simulink model "C28069_LLC_ePWM_V8_230307_PhaeShiftWorking"  (R2022b)
settings: Solver=FixedStepAuto  StartTime=0.0  StopTime=10  RelTol=1e-3  EnableMultiTasking=on
model workspace (MAT data in the model file):
  Comp_DAC = 512
undefined symbols (not defined in the file or in its folder): Down, GPTRIP1SEL, GPTRIP2SEL, PWM_Control, PWM_Gen, PWM_Gen1, SCI_A_Transmit, SCI_A_Transmit_Current_Suffix, SCI_A_Transmit_Duty_Suffix, SCI_A_Transmit_Freq_Suffix, SCI_A_Transmit_OVPFlag_Suffix, SCI_A_Transmit_PFC_Suffix, SCI_A_Transmit_SS_Suffix, SCI_A_Transmit_TBPHS_Suffix, SCI_A_Transmit_VADC_Suffix, SCI_A_Transmit_VAvg_Suffix, SCI_A_Transmit_VBAT_Suffix, SCI_A_Transmit_VBATRef_Suffix, SCI_A_Transmit_Vo_Suffix, TZ1, TZ2, u1, Up
libraries: c2802xlib x92, c280xlib x39, simulink x36, c2000lib x1
(part 15 of 18)

== system C28069_LLC_ePWM_V8_230307_PhaeShiftWorking/Softstart @5kHz/GetADC, FaultProtection, SoftStart  @5KHz/UpdatePWM/Frequency Update/Simulink Function1 ==
  note: Original
  note: Frequency Input Selection
  note: Control CMPA/B to Zero
      | When the input is <1KHz
      | (To switch off ePWM)
  note: Fixing deadtime to 250ns
  note: Added Trigger
  PWM_Gen : TriggerPort  TriggerType=function-call  IsSimulinkFunction=on  FunctionName=PWM_Gen  FunctionVisibility=scoped  VariantControl=(inherit)
  CMPA : Display
  CMPA1 : Display
  CMPB : Display
  CMPB1 : Display
  Constant : Constant  Value=100
  Constant1 : Constant
  Constant2 : Constant  Value=0
  Constant3 : Constant  Value=50
  Constant4 : Constant
  Dead time (%) : Display
  Dead time (sec) : Constant  Value=250E-9
  Divide : Product  Inputs=*/
  Gain1 : Gain  Gain=1000
  Gain2 : Gain  Gain=100
  Product{1..4} (4 alike) : Product
  Subsystem1 : Subsystem
  Subtract : Sum  Inputs=+-
  Switch : Switch  Criteria=u2 > Threshold  Threshold=1  SaturateOnIntegerOverflow=off  InputSameDT=off
  Switch1 : Switch  Criteria=u2 > Threshold  OutDataTypeStr=double  SaturateOnIntegerOverflow=off  InputSameDT=off
  TBPRD : Display
  ePWM1 : c2802xlib/ePWM  PwmType=C2000  useModule=ePWM6  ePWMxLINKTBPRD=Not Linked  periodUnits=Clock cycles  timerSource=Input port  timerPeriod_clk=294  timerPeriod_sec=0.0001  tbshadow=Counter equals to zero  countingMode=Up-Down  phaseActiveEnable=Disable  phaseDirection=Count down after sync  phaseActive=0  synchronizationEnable=off  dcaevt1Sync=off  dcbevt1Sync=off  synchronizationOption=Disable  dcbevt1SyncOut=off  dcaevt1SyncOut=off  cmpdSyncOut=off  cmpcSyncOut=off  cmpbSyncOut=off  zeroSyncOut=off  swfSyncOut=off  perSynchronizationOption=Counter equals to period (CTR=PRD)  clockPrescale=1  HSclockPrescale=1  enswap=off  ePWMxAStatus=on  ePWMxAactionLogic1=Do nothing  ePWMxAactionLogic2=Do nothing  ePWMxAactionLogic3=Set  ePWMxAactionLogic4=Do nothing  ePWMxAactionLogic5=Clear  ePWMxAactionLogic6=Do nothing  ePWMxACSFenable=off  ePWMxACSFvalue=Forcing disable  ePWMxASFreload=Zero  ePWMxBStatus=on  ePWMxBactionLogic1=Do nothing  ePWMxBactionLogic2=Do nothing  ePWMxBactionLogic3=Do nothing  ePWMxBactionLogic4=Clear  ePWMxBactionLogic5=Do nothing  ePWMxBactionLogic6=Set  ePWMxBCSFenable=off  ePWMxBCSFvalue=Forcing disable  ePWMxBSFreload=Zero  ePWNxBOutWay=off  ePWMxLINKCMPA=Not Linked  CMPAUnits=Clock cycles  CMPASource=Input port  CMPAValue_per=50  CMPAValue_clk=0  enCMPAshadow=Counter equals to zero (CTR=Zero)  ePWMxLINKCMPB=Not Linked  CMPBUnits=Clock cycles  CMPBSource=Input port  CMPBValue_per=50  CMPBValue_clk=0  enCMPBshadow=Counter equals to zero (CTR=Zero)  ePWMxLINKCMPC=Not Linked  CMPCUnits=Clock cycles  CMPCSource=Specify via dialog  CMPCValue_per=50  CMPCValue_clk=32000  enCMPCshadow=Counter equals to zero (CTR=Zero)  ePWMxLINKCMPD=Not Linked  CMPDUnits=Clock cycles  CMPDSource=Specify via dialog  CMPDValue_per=50  CMPDValue_clk=32000  enCMPDshadow=Counter equals to zero (CTR=Zero)  enableDBePWMxA=off  enableDBePWMxB=off  enhalfcycle=off  DBpolarity=Active high complementary (AHC)  DBedgeDelay=Positive  DBSource_ePWMxA=ePWMxA  DBSource_ePWMxB=ePWMxA  DBPeriodUnits=Clock cycles  DBperiodSource=Input port  REDperiod=10  FEDperiod=10  REDperiod_sec=0  FEDperiod_sec=0  LoadModeDBRED=Immediate without using shadow  LoadModeDBFED=Immediate without using shadow  adcstartModuleA=off  adcrequestEventA=First event  adcstartEventA=Counter equals to zero (CTR=Zero)  adcstartEventA_type2=Digital Compare Module A Event 1 start of conversion (DCAEVT1.soc)  adcstartModuleB=off  adcrequestEventB=First event  adcstartEventB=Counter equals to zero (CTR=Zero)  adcstartEventB_type2=Counter equals to zero (CTR=Zero)  intEn=off  intPrd=First event  intSel=Counter equals to zero (CTR=Zero)  intSel_type2=Counter equals to zero (CTR=Zero)  hrpe=off  enHRPWM=off  HRPWM_LoadMode=Counter equals to period (CTR=PRD)  HRPWM_CTLMode=Duty or Period control mode  HRPWM_EDGMode=Both edge  hrpeb=off  enHRPWMB=off  HRPWM_LoadModeB=Counter equals to zero (CTR=ZERO)  HRPWM_CTLModeB=Duty or Period control mode  HRPWM_EDGModeB=Both edge  enHRDBRED=off  enHRDBFED=off  enSFO=on  enautoconv=on  chopperEnable=off  chopperFrequency=1  chopperFirstwidth=1  chopperDuty=12.5%  tripZonesource=Specify via dialog  tzselOSHT1=off  tzselOSHT2=off  tzselOSHT3=off  tzselOSHDCAEV1=off  tzselOSHDCBEV1=off  tzselCBC1=off  tzselCBC2=off  tzselCBC3=off  tzselCBCDCAEV2=off  tzselCBCDCBEV2=off  tzselOSHT4=off  tzselOSHT5=off  tzselOSHT6=off  tzselCBC4=off  tzselCBC5=off  tzselCBC6=off  enTzOstIntr=off  enTzCbcIntr=off  enTzDCAEVT1Intr=off  enTzDCAEVT2Intr=off  enTzDCBEVT1Intr=off  enTzDCBEVT2Intr=off  ePWMxAforced=No action  ePWMxBforced=No action  DCAEVT1forced=Low  DCBEVT1forced=Low  DCAEVT2forced=No action  DCBEVT2forced=No action  dcah=COMP1OUT input  dcal=Trip Zone 1 input (TZ1)  dcbh=COMP1OUT input  dcbl=Trip Zone 1 input (TZ1)  dcah_type2=GPTRIP1SEL/(TZ1)  dcal_type2=GPTRIP2SEL/(TZ2)  dcbh_type2=GPTRIP1SEL/(TZ1)  dcbl_type2=GPTRIP2SEL/(TZ2)  gendcaevt1=DCAH=high and DCAL=don't care  gendcaevt2=Event disabled  gendcbevt1=DCBH=high and DCBL=don't care  gendcbevt2=Event disabled  dcaevt1src=DCAEVT1 with sync  dcaevt2src=DCAEVT2 with sync  dcbevt1src=DCBEVT1 with sync  dcbevt2src=DCBEVT2 with sync  pulsesel=Counter equals to zero (CTR=Zero)  blankinv=off  blankoffset=0  blankwidth=0  evsrcsel=Filtered version of DCAEVT1 (DCAEVT1FILT)  encape=off
      settings: LibrarySourceBlock=c2806xlib/ePWM
  ePWM4 : c2802xlib/ePWM  PwmType=C2000  useModule=ePWM5  ePWMxLINKTBPRD=Not Linked  periodUnits=Clock cycles  timerSource=Input port  timerPeriod_clk=294  timerPeriod_sec=0.0001  tbshadow=Counter equals to zero  countingMode=Up-Down  phaseActiveEnable=Disable  phaseDirection=Count down after sync  phaseActive=0  synchronizationEnable=off  dcaevt1Sync=off  dcbevt1Sync=off  synchronizationOption=Disable  dcbevt1SyncOut=off  dcaevt1SyncOut=off  cmpdSyncOut=off  cmpcSyncOut=off  cmpbSyncOut=off  zeroSyncOut=off  swfSyncOut=off  perSynchronizationOption=Counter equals to period (CTR=PRD)  clockPrescale=1  HSclockPrescale=1  enswap=off  ePWMxAStatus=on  ePWMxAactionLogic1=Do nothing  ePWMxAactionLogic2=Do nothing  ePWMxAactionLogic3=Set  ePWMxAactionLogic4=Do nothing  ePWMxAactionLogic5=Clear  ePWMxAactionLogic6=Do nothing  ePWMxACSFenable=off  ePWMxACSFvalue=Forcing disable  ePWMxASFreload=Zero  ePWMxBStatus=on  ePWMxBactionLogic1=Do nothing  ePWMxBactionLogic2=Do nothing  ePWMxBactionLogic3=Do nothing  ePWMxBactionLogic4=Clear  ePWMxBactionLogic5=Do nothing  ePWMxBactionLogic6=Set  ePWMxBCSFenable=off  ePWMxBCSFvalue=Forcing disable  ePWMxBSFreload=Zero  ePWNxBOutWay=off  ePWMxLINKCMPA=Not Linked  CMPAUnits=Clock cycles  CMPASource=Input port  CMPAValue_per=50  CMPAValue_clk=0  enCMPAshadow=Counter equals to zero (CTR=Zero)  ePWMxLINKCMPB=Not Linked  CMPBUnits=Clock cycles  CMPBSource=Input port  CMPBValue_per=50  CMPBValue_clk=0  enCMPBshadow=Counter equals to zero (CTR=Zero)  ePWMxLINKCMPC=Not Linked  CMPCUnits=Clock cycles  CMPCSource=Specify via dialog  CMPCValue_per=50  CMPCValue_clk=32000  enCMPCshadow=Counter equals to zero (CTR=Zero)  ePWMxLINKCMPD=Not Linked  CMPDUnits=Clock cycles  CMPDSource=Specify via dialog  CMPDValue_per=50  CMPDValue_clk=32000  enCMPDshadow=Counter equals to zero (CTR=Zero)  enableDBePWMxA=off  enableDBePWMxB=off  enhalfcycle=off  DBpolarity=Active high complementary (AHC)  DBedgeDelay=Positive  DBSource_ePWMxA=ePWMxA  DBSource_ePWMxB=ePWMxA  DBPeriodUnits=Clock cycles  DBperiodSource=Input port  REDperiod=10  FEDperiod=10  REDperiod_sec=0  FEDperiod_sec=0  LoadModeDBRED=Immediate without using shadow  LoadModeDBFED=Immediate without using shadow  adcstartModuleA=on  adcrequestEventA=First event  adcstartEventA=Counter equals to zero (CTR=Zero)  adcstartEventA_type2=Digital Compare Module A Event 1 start of conversion (DCAEVT1.soc)  adcstartModuleB=off  adcrequestEventB=First event  adcstartEventB=Counter equals to zero (CTR=Zero)  adcstartEventB_type2=Counter equals to zero (CTR=Zero)  intEn=on  intPrd=First event  intSel=Counter equals to zero (CTR=Zero)  intSel_type2=Counter equals to zero (CTR=Zero)  hrpe=off  enHRPWM=off  HRPWM_LoadMode=Counter equals to period (CTR=PRD)  HRPWM_CTLMode=Duty or Period control mode  HRPWM_EDGMode=Both edge  hrpeb=off  enHRPWMB=off  HRPWM_LoadModeB=Counter equals to zero (CTR=ZERO)  HRPWM_CTLModeB=Duty or Period control mode  HRPWM_EDGModeB=Both edge  enHRDBRED=off  enHRDBFED=off  enSFO=on  enautoconv=on  chopperEnable=off  chopperFrequency=1  chopperFirstwidth=1  chopperDuty=12.5%  tripZonesource=Specify via dialog  tzselOSHT1=off  tzselOSHT2=off  tzselOSHT3=off  tzselOSHDCAEV1=off  tzselOSHDCBEV1=off  tzselCBC1=off  tzselCBC2=off  tzselCBC3=off  tzselCBCDCAEV2=off  tzselCBCDCBEV2=off  tzselOSHT4=off  tzselOSHT5=off  tzselOSHT6=off  tzselCBC4=off  tzselCBC5=off  tzselCBC6=off  enTzOstIntr=off  enTzCbcIntr=off  enTzDCAEVT1Intr=off  enTzDCAEVT2Intr=off  enTzDCBEVT1Intr=off  enTzDCBEVT2Intr=off  ePWMxAforced=No action  ePWMxBforced=No action  DCAEVT1forced=Low  DCBEVT1forced=Low  DCAEVT2forced=No action  DCBEVT2forced=No action  dcah=COMP1OUT input  dcal=Trip Zone 1 input (TZ1)  dcbh=COMP1OUT input  dcbl=Trip Zone 1 input (TZ1)  dcah_type2=GPTRIP1SEL/(TZ1)  dcal_type2=GPTRIP2SEL/(TZ2)  dcbh_type2=GPTRIP1SEL/(TZ1)  dcbl_type2=GPTRIP2SEL/(TZ2)  gendcaevt1=DCAH=high and DCAL=don't care  gendcaevt2=Event disabled  gendcbevt1=DCBH=high and DCBL=don't care  gendcbevt2=Event disabled  dcaevt1src=DCAEVT1 with sync  dcaevt2src=DCAEVT2 with sync  dcbevt1src=DCBEVT1 with sync  dcbevt2src=DCBEVT2 with sync  pulsesel=Counter equals to zero (CTR=Zero)  blankinv=off  blankoffset=0  blankwidth=0  evsrcsel=Filtered version of DCAEVT1 (DCAEVT1FILT)  encape=off
      settings: LibrarySourceBlock=c2806xlib/ePWM
  original : c2802xlib/ePWM  Commented=on  PwmType=C2000  useModule=ePWM6  ePWMxLINKTBPRD=Not Linked  periodUnits=Clock cycles  timerSource=Input port  timerPeriod_clk=294  timerPeriod_sec=0.0001  tbshadow=Counter equals to zero  countingMode=Up-Down  phaseActiveEnable=Disable  phaseDirection=Count down after sync  phaseActive=0  synchronizationEnable=off  dcaevt1Sync=off  dcbevt1Sync=off  synchronizationOption=Disable  dcbevt1SyncOut=off  dcaevt1SyncOut=off  cmpdSyncOut=off  cmpcSyncOut=off  cmpbSyncOut=off  zeroSyncOut=off  swfSyncOut=off  perSynchronizationOption=Counter equals to period (CTR=PRD)  clockPrescale=1  HSclockPrescale=1  enswap=off  ePWMxAStatus=on  ePWMxAactionLogic1=Do nothing  ePWMxAactionLogic2=Do nothing  ePWMxAactionLogic3=Set  ePWMxAactionLogic4=Do nothing  ePWMxAactionLogic5=Clear  ePWMxAactionLogic6=Do nothing  ePWMxACSFenable=off  ePWMxACSFvalue=Forcing disable  ePWMxASFreload=Zero  ePWMxBStatus=on  ePWMxBactionLogic1=Do nothing  ePWMxBactionLogic2=Do nothing  ePWMxBactionLogic3=Do nothing  ePWMxBactionLogic4=Clear  ePWMxBactionLogic5=Do nothing  ePWMxBactionLogic6=Set  ePWMxBCSFenable=off  ePWMxBCSFvalue=Forcing disable  ePWMxBSFreload=Zero  ePWNxBOutWay=off  ePWMxLINKCMPA=Not Linked  CMPAUnits=Clock cycles  CMPASource=Input port  CMPAValue_per=50  CMPAValue_clk=12  enCMPAshadow=Counter equals to zero (CTR=Zero)  ePWMxLINKCMPB=Not Linked  CMPBUnits=Clock cycles  CMPBSource=Input port  CMPBValue_per=50  CMPBValue_clk=283  enCMPBshadow=Counter equals to zero (CTR=Zero)  ePWMxLINKCMPC=Not Linked  CMPCUnits=Clock cycles  CMPCSource=Specify via dialog  CMPCValue_per=50  CMPCValue_clk=32000  enCMPCshadow=Counter equals to zero (CTR=Zero)  ePWMxLINKCMPD=Not Linked  CMPDUnits=Clock cycles  CMPDSource=Specify via dialog  CMPDValue_per=50  CMPDValue_clk=32000  enCMPDshadow=Counter equals to zero (CTR=Zero)  enableDBePWMxA=off  enableDBePWMxB=off  enhalfcycle=off  DBpolarity=Active high complementary (AHC)  DBedgeDelay=Positive  DBSource_ePWMxA=ePWMxA  DBSource_ePWMxB=ePWMxA  DBPeriodUnits=Clock cycles  DBperiodSource=Input port  REDperiod=10  FEDperiod=10  REDperiod_sec=0  FEDperiod_sec=0  LoadModeDBRED=Immediate without using shadow  LoadModeDBFED=Immediate without using shadow  adcstartModuleA=off  adcrequestEventA=First event  adcstartEventA=Counter equals to zero (CTR=Zero)  adcstartEventA_type2=Digital Compare Module A Event 1 start of conversion (DCAEVT1.soc)  adcstartModuleB=off  adcrequestEventB=First event  adcstartEventB=Counter equals to zero (CTR=Zero)  adcstartEventB_type2=Counter equals to zero (CTR=Zero)  intEn=off  intPrd=First event  intSel=Counter equals to zero (CTR=Zero)  intSel_type2=Counter equals to zero (CTR=Zero)  hrpe=off  enHRPWM=off  HRPWM_LoadMode=Counter equals to period (CTR=PRD)  HRPWM_CTLMode=Duty or Period control mode  HRPWM_EDGMode=Both edge  hrpeb=off  enHRPWMB=off  HRPWM_LoadModeB=Counter equals to zero (CTR=ZERO)  HRPWM_CTLModeB=Duty or Period control mode  HRPWM_EDGModeB=Both edge  enHRDBRED=off  enHRDBFED=off  enSFO=on  enautoconv=on  chopperEnable=off  chopperFrequency=1  chopperFirstwidth=1  chopperDuty=12.5%  tripZonesource=Specify via dialog  tzselOSHT1=off  tzselOSHT2=off  tzselOSHT3=off  tzselOSHDCAEV1=off  tzselOSHDCBEV1=off  tzselCBC1=off  tzselCBC2=off  tzselCBC3=off  tzselCBCDCAEV2=off  tzselCBCDCBEV2=off  tzselOSHT4=off  tzselOSHT5=off  tzselOSHT6=off  tzselCBC4=off  tzselCBC5=off  tzselCBC6=off  enTzOstIntr=off  enTzCbcIntr=off  enTzDCAEVT1Intr=off  enTzDCAEVT2Intr=off  enTzDCBEVT1Intr=off  enTzDCBEVT2Intr=off  ePWMxAforced=No action  ePWMxBforced=No action  DCAEVT1forced=Low  DCBEVT1forced=Low  DCAEVT2forced=No action  DCBEVT2forced=No action  dcah=COMP1OUT input  dcal=Trip Zone 1 input (TZ1)  dcbh=COMP1OUT input  dcbl=Trip Zone 1 input (TZ1)  dcah_type2=GPTRIP1SEL/(TZ1)  dcal_type2=GPTRIP2SEL/(TZ2)  dcbh_type2=GPTRIP1SEL/(TZ1)  dcbl_type2=GPTRIP2SEL/(TZ2)  gendcaevt1=DCAH=high and DCAL=don't care  gendcaevt2=Event disabled  gendcbevt1=DCBH=high and DCBL=don't care  gendcbevt2=Event disabled  dcaevt1src=DCAEVT1 with sync  dcaevt2src=DCAEVT2 with sync  dcbevt1src=DCBEVT1 with sync  dcbevt2src=DCBEVT2 with sync  pulsesel=Counter equals to zero (CTR=Zero)  blankinv=off  blankoffset=0  blankwidth=0  evsrcsel=Filtered version of DCAEVT1 (DCAEVT1FILT)  encape=off
      settings: LibrarySourceBlock=c2806xlib/ePWM
  u : ArgIn  DisableCoverage=on  ArgumentName=u
  wires:
  Constant4/1 -> Switch1/3
  Product4/1 -> ePWM1/3, ePWM4/3, CMPB1/1
  Product3/1 -> CMPA1/1, ePWM4/2, ePWM1/2
  Switch/1 -> Product4/2, Product3/2
  Constant2/1 -> Switch/3
  Constant1/1 -> Switch/1
  Dead time (sec)/1 -> Product1/2
  Gain1/1 -> Product1/1
  Subsystem1/1(Out1) -> TBPRD/1, ePWM1/1, ePWM4/1, Subtract/1, Product2/1
  Product1/1 -> Gain2/1
  Subtract/1 -> CMPB/1, Product4/1
  Constant/1 -> Divide/2
  Product2/1 -> CMPA/1, Product3/1, Subtract/2
  Divide/1 -> Product2/2
  Constant3/1 -> Subsystem1/2(Duty(%))
  u/1 -> Switch1/2, Switch1/1
  Switch1/1 -> Gain1/1, Switch/2, Subsystem1/1(Frequency(kHz))
  Gain2/1 -> Dead time (%)/1, Divide/1

== system C28069_LLC_ePWM_V8_230307_PhaeShiftWorking/Softstart @5kHz/GetADC, FaultProtection, SoftStart  @5KHz/UpdatePWM/Frequency Update/Simulink Function2 ==
  note: Original
  note: Frequency Input Selection
  note: Control CMPA/B to Zero
      | When the input is <1KHz
      | (To switch off ePWM)
  note: Fixing deadtime to 250ns
  note: Added Trigger
  PWM_Gen1 : TriggerPort  TriggerType=function-call  IsSimulinkFunction=on  FunctionName=PWM_Gen1  FunctionVisibility=scoped  VariantControl=(inherit)
  CMPA : Display
  CMPA1 : Display
  CMPB : Display
  CMPB1 : Display
  Constant : Constant  Value=100
  Constant1 : Constant
  Constant2 : Constant  Value=0
  Constant3 : Constant  Value=50
  Constant4 : Constant
  Dead time (%) : Display
  Dead time (sec) : Constant  Value=250E-9
  Divide : Product  Inputs=*/
  Gain1 : Gain  Gain=1000
  Gain2 : Gain  Commented=on  Gain=100
  Product1 : Product  Inputs=3
  Product2 : Product
  Product3 : Product
  Product4 : Product
  Subsystem1 : Subsystem
  Subtract : Sum  Inputs=+-
  Switch : Switch  Criteria=u2 > Threshold  Threshold=1  SaturateOnIntegerOverflow=off  InputSameDT=off
  Switch1 : Switch  Criteria=u2 > Threshold  SaturateOnIntegerOverflow=off  InputSameDT=off
  TBPRD : Display
  ePWM1 : c2802xlib/ePWM  PwmType=C2000  useModule=ePWM6  ePWMxLINKTBPRD=Not Linked  periodUnits=Clock cycles  timerSource=Input port  timerPeriod_clk=294  timerPeriod_sec=0.0001  tbshadow=Counter equals to zero  countingMode=Up-Down  phaseActiveEnable=Disable  phaseDirection=Count down after sync  phaseActive=0  synchronizationEnable=off  dcaevt1Sync=off  dcbevt1Sync=off  synchronizationOption=Disable  dcbevt1SyncOut=off  dcaevt1SyncOut=off  cmpdSyncOut=off  cmpcSyncOut=off  cmpbSyncOut=off  zeroSyncOut=off  swfSyncOut=off  perSynchronizationOption=Counter equals to period (CTR=PRD)  clockPrescale=1  HSclockPrescale=1  enswap=off  ePWMxAStatus=on  ePWMxAactionLogic1=Do nothing  ePWMxAactionLogic2=Do nothing  ePWMxAactionLogic3=Set  ePWMxAactionLogic4=Do nothing  ePWMxAactionLogic5=Clear  ePWMxAactionLogic6=Do nothing  ePWMxACSFenable=off  ePWMxACSFvalue=Forcing disable  ePWMxASFreload=Zero  ePWMxBStatus=on  ePWMxBactionLogic1=Do nothing  ePWMxBactionLogic2=Do nothing  ePWMxBactionLogic3=Do nothing  ePWMxBactionLogic4=Clear  ePWMxBactionLogic5=Do nothing  ePWMxBactionLogic6=Set  ePWMxBCSFenable=off  ePWMxBCSFvalue=Forcing disable  ePWMxBSFreload=Zero  ePWNxBOutWay=off  ePWMxLINKCMPA=Not Linked  CMPAUnits=Clock cycles  CMPASource=Input port  CMPAValue_per=50  CMPAValue_clk=12  enCMPAshadow=Counter equals to zero (CTR=Zero)  ePWMxLINKCMPB=Not Linked  CMPBUnits=Clock cycles  CMPBSource=Input port  CMPBValue_per=50  CMPBValue_clk=283  enCMPBshadow=Counter equals to zero (CTR=Zero)  ePWMxLINKCMPC=Not Linked  CMPCUnits=Clock cycles  CMPCSource=Specify via dialog  CMPCValue_per=50  CMPCValue_clk=32000  enCMPCshadow=Counter equals to zero (CTR=Zero)  ePWMxLINKCMPD=Not Linked  CMPDUnits=Clock cycles  CMPDSource=Specify via dialog  CMPDValue_per=50  CMPDValue_clk=32000  enCMPDshadow=Counter equals to zero (CTR=Zero)  enableDBePWMxA=off  enableDBePWMxB=off  enhalfcycle=off  DBpolarity=Active high complementary (AHC)  DBedgeDelay=Positive  DBSource_ePWMxA=ePWMxA  DBSource_ePWMxB=ePWMxA  DBPeriodUnits=Clock cycles  DBperiodSource=Input port  REDperiod=10  FEDperiod=10  REDperiod_sec=0  FEDperiod_sec=0  LoadModeDBRED=Immediate without using shadow  LoadModeDBFED=Immediate without using shadow  adcstartModuleA=off  adcrequestEventA=First event  adcstartEventA=Counter equals to zero (CTR=Zero)  adcstartEventA_type2=Digital Compare Module A Event 1 start of conversion (DCAEVT1.soc)  adcstartModuleB=off  adcrequestEventB=First event  adcstartEventB=Counter equals to zero (CTR=Zero)  adcstartEventB_type2=Counter equals to zero (CTR=Zero)  intEn=off  intPrd=First event  intSel=Counter equals to zero (CTR=Zero)  intSel_type2=Counter equals to zero (CTR=Zero)  hrpe=off  enHRPWM=off  HRPWM_LoadMode=Counter equals to period (CTR=PRD)  HRPWM_CTLMode=Duty or Period control mode  HRPWM_EDGMode=Both edge  hrpeb=off  enHRPWMB=off  HRPWM_LoadModeB=Counter equals to zero (CTR=ZERO)  HRPWM_CTLModeB=Duty or Period control mode  HRPWM_EDGModeB=Both edge  enHRDBRED=off  enHRDBFED=off  enSFO=on  enautoconv=on  chopperEnable=off  chopperFrequency=1  chopperFirstwidth=1  chopperDuty=12.5%  tripZonesource=Specify via dialog  tzselOSHT1=off  tzselOSHT2=off  tzselOSHT3=off  tzselOSHDCAEV1=off  tzselOSHDCBEV1=off  tzselCBC1=off  tzselCBC2=off  tzselCBC3=off  tzselCBCDCAEV2=off  tzselCBCDCBEV2=off  tzselOSHT4=off  tzselOSHT5=off  tzselOSHT6=off  tzselCBC4=off  tzselCBC5=off  tzselCBC6=off  enTzOstIntr=off  enTzCbcIntr=off  enTzDCAEVT1Intr=off  enTzDCAEVT2Intr=off  enTzDCBEVT1Intr=off  enTzDCBEVT2Intr=off  ePWMxAforced=No action  ePWMxBforced=No action  DCAEVT1forced=Low  DCBEVT1forced=Low  DCAEVT2forced=No action  DCBEVT2forced=No action  dcah=COMP1OUT input  dcal=Trip Zone 1 input (TZ1)  dcbh=COMP1OUT input  dcbl=Trip Zone 1 input (TZ1)  dcah_type2=GPTRIP1SEL/(TZ1)  dcal_type2=GPTRIP2SEL/(TZ2)  dcbh_type2=GPTRIP1SEL/(TZ1)  dcbl_type2=GPTRIP2SEL/(TZ2)  gendcaevt1=DCAH=high and DCAL=don't care  gendcaevt2=Event disabled  gendcbevt1=DCBH=high and DCBL=don't care  gendcbevt2=Event disabled  dcaevt1src=DCAEVT1 with sync  dcaevt2src=DCAEVT2 with sync  dcbevt1src=DCBEVT1 with sync  dcbevt2src=DCBEVT2 with sync  pulsesel=Counter equals to zero (CTR=Zero)  blankinv=off  blankoffset=0  blankwidth=0  evsrcsel=Filtered version of DCAEVT1 (DCAEVT1FILT)  encape=off
      settings: LibrarySourceBlock=c2806xlib/ePWM
  ePWM4 : c2802xlib/ePWM  PwmType=C2000  useModule=ePWM5  ePWMxLINKTBPRD=Not Linked  periodUnits=Clock cycles  timerSource=Input port  timerPeriod_clk=294  timerPeriod_sec=0.0001  tbshadow=Counter equals to zero  countingMode=Up-Down  phaseActiveEnable=Disable  phaseDirection=Count down after sync  phaseActive=0  synchronizationEnable=off  dcaevt1Sync=off  dcbevt1Sync=off  synchronizationOption=Disable  dcbevt1SyncOut=off  dcaevt1SyncOut=off  cmpdSyncOut=off  cmpcSyncOut=off  cmpbSyncOut=off  zeroSyncOut=off  swfSyncOut=off  perSynchronizationOption=Counter equals to period (CTR=PRD)  clockPrescale=1  HSclockPrescale=1  enswap=off  ePWMxAStatus=on  ePWMxAactionLogic1=Do nothing  ePWMxAactionLogic2=Do nothing  ePWMxAactionLogic3=Set  ePWMxAactionLogic4=Do nothing  ePWMxAactionLogic5=Clear  ePWMxAactionLogic6=Do nothing  ePWMxACSFenable=off  ePWMxACSFvalue=Forcing disable  ePWMxASFreload=Zero  ePWMxBStatus=on  ePWMxBactionLogic1=Do nothing  ePWMxBactionLogic2=Do nothing  ePWMxBactionLogic3=Do nothing  ePWMxBactionLogic4=Clear  ePWMxBactionLogic5=Do nothing  ePWMxBactionLogic6=Set  ePWMxBCSFenable=off  ePWMxBCSFvalue=Forcing disable  ePWMxBSFreload=Zero  ePWNxBOutWay=off  ePWMxLINKCMPA=Not Linked  CMPAUnits=Clock cycles  CMPASource=Input port  CMPAValue_per=50  CMPAValue_clk=12  enCMPAshadow=Counter equals to zero (CTR=Zero)  ePWMxLINKCMPB=Not Linked  CMPBUnits=Clock cycles  CMPBSource=Input port  CMPBValue_per=50  CMPBValue_clk=283  enCMPBshadow=Counter equals to zero (CTR=Zero)  ePWMxLINKCMPC=Not Linked  CMPCUnits=Clock cycles  CMPCSource=Specify via dialog  CMPCValue_per=50  CMPCValue_clk=32000  enCMPCshadow=Counter equals to zero (CTR=Zero)  ePWMxLINKCMPD=Not Linked  CMPDUnits=Clock cycles  CMPDSource=Specify via dialog  CMPDValue_per=50  CMPDValue_clk=32000  enCMPDshadow=Counter equals to zero (CTR=Zero)  enableDBePWMxA=off  enableDBePWMxB=off  enhalfcycle=off  DBpolarity=Active high complementary (AHC)  DBedgeDelay=Positive  DBSource_ePWMxA=ePWMxA  DBSource_ePWMxB=ePWMxA  DBPeriodUnits=Clock cycles  DBperiodSource=Input port  REDperiod=10  FEDperiod=10  REDperiod_sec=0  FEDperiod_sec=0  LoadModeDBRED=Immediate without using shadow  LoadModeDBFED=Immediate without using shadow  adcstartModuleA=on  adcrequestEventA=First event  adcstartEventA=Counter equals to zero (CTR=Zero)  adcstartEventA_type2=Digital Compare Module A Event 1 start of conversion (DCAEVT1.soc)  adcstartModuleB=off  adcrequestEventB=First event  adcstartEventB=Counter equals to zero (CTR=Zero)  adcstartEventB_type2=Counter equals to zero (CTR=Zero)  intEn=on  intPrd=First event  intSel=Counter equals to zero (CTR=Zero)  intSel_type2=Counter equals to zero (CTR=Zero)  hrpe=off  enHRPWM=off  HRPWM_LoadMode=Counter equals to period (CTR=PRD)  HRPWM_CTLMode=Duty or Period control mode  HRPWM_EDGMode=Both edge  hrpeb=off  enHRPWMB=off  HRPWM_LoadModeB=Counter equals to zero (CTR=ZERO)  HRPWM_CTLModeB=Duty or Period control mode  HRPWM_EDGModeB=Both edge  enHRDBRED=off  enHRDBFED=off  enSFO=on  enautoconv=on  chopperEnable=off  chopperFrequency=1  chopperFirstwidth=1  chopperDuty=12.5%  tripZonesource=Specify via dialog  tzselOSHT1=off  tzselOSHT2=off  tzselOSHT3=off  tzselOSHDCAEV1=off  tzselOSHDCBEV1=off  tzselCBC1=off  tzselCBC2=off  tzselCBC3=off  tzselCBCDCAEV2=off  tzselCBCDCBEV2=off  tzselOSHT4=off  tzselOSHT5=off  tzselOSHT6=off  tzselCBC4=off  tzselCBC5=off  tzselCBC6=off  enTzOstIntr=off  enTzCbcIntr=off  enTzDCAEVT1Intr=off  enTzDCAEVT2Intr=off  enTzDCBEVT1Intr=off  enTzDCBEVT2Intr=off  ePWMxAforced=No action  ePWMxBforced=No action  DCAEVT1forced=Low  DCBEVT1forced=Low  DCAEVT2forced=No action  DCBEVT2forced=No action  dcah=COMP1OUT input  dcal=Trip Zone 1 input (TZ1)  dcbh=COMP1OUT input  dcbl=Trip Zone 1 input (TZ1)  dcah_type2=GPTRIP1SEL/(TZ1)  dcal_type2=GPTRIP2SEL/(TZ2)  dcbh_type2=GPTRIP1SEL/(TZ1)  dcbl_type2=GPTRIP2SEL/(TZ2)  gendcaevt1=DCAH=high and DCAL=don't care  gendcaevt2=Event disabled  gendcbevt1=DCBH=high and DCBL=don't care  gendcbevt2=Event disabled  dcaevt1src=DCAEVT1 with sync  dcaevt2src=DCAEVT2 with sync  dcbevt1src=DCBEVT1 with sync  dcbevt2src=DCBEVT2 with sync  pulsesel=Counter equals to zero (CTR=Zero)  blankinv=off  blankoffset=0  blankwidth=0  evsrcsel=Filtered version of DCAEVT1 (DCAEVT1FILT)  encape=off
      settings: LibrarySourceBlock=c2806xlib/ePWM
  u : ArgIn  DisableCoverage=on  OutDataTypeStr=uint16  ArgumentName=u
  u1 : ArgIn  DisableCoverage=on  Port=2  OutDataTypeStr=uint16  ArgumentName=u1
  wires:
  Constant4/1 -> Switch1/3
  Product4/1 -> ePWM1/3, ePWM4/3, CMPB1/1
  Product3/1 -> CMPA1/1, ePWM4/2, ePWM1/2
  Switch/1 -> Product4/2, Product3/2
  Constant2/1 -> Switch/3
  Constant1/1 -> Switch/1
  Dead time (sec)/1 -> Product1/2
  Gain1/1 -> Product1/1
  Subsystem1/1(Out1) -> TBPRD/1, ePWM1/1, ePWM4/1, Subtract/1, Product2/1
  Product1/1 -> Dead time (%)/1, Divide/1
  Subtract/1 -> CMPB/1, Product4/1
  Constant/1 -> Divide/2
  Product2/1 -> CMPA/1, Product3/1, Subtract/2
  Divide/1 -> Product2/2
  Constant3/1 -> Subsystem1/2(Duty(%))
  u/1 -> Switch1/2, Switch1/1
  Switch1/1 -> Gain1/1, Switch/2, Subsystem1/1(Frequency(kHz))
  u1/1 -> Product1/3

== system C28069_LLC_ePWM_V8_230307_PhaeShiftWorking/Softstart @5kHz/GetADC, FaultProtection, SoftStart  @5KHz/UpdatePWM/Frequency Update/Simulink Function1/Subsystem1 ==
  Frequency(kHz) : Inport  OutDataTypeStr=double
  Duty(%) : Inport  Port=2
  Constant1 : Constant  Value=90E6
  Divide : Product  Inputs=*/  RndMeth=Zero  SaturateOnIntegerOverflow=on
  Gain : Gain  Gain=1000
  Gain1 : Gain  Gain=1/100
  Gain2 : Gain  Gain=0.5
  Product : Product
  Product1 : Product
  Up-Down Counter : Constant  Value=2
  Out1 : Outport
  Out2 : Outport  Port=2
  Out3 : Outport  Port=3
  wires:
  Gain2/1 -> Out3/1
  Gain1/1 -> Product1/2
  Product1/1 -> Gain2/1, Out2/1
  Duty(%)/1 -> Gain1/1
  Divide/1 -> Out1/1, Product1/1
  Constant1/1 -> Divide/1
  Frequency(kHz)/1 -> Gain/1
  Product/1 -> Divide/2
  Gain/1 -> Product/1
  Up-Down Counter/1 -> Product/2

== system C28069_LLC_ePWM_V8_230307_PhaeShiftWorking/Softstart @5kHz/GetADC, FaultProtection, SoftStart  @5KHz/UpdatePWM/Frequency Update/Simulink Function2/Subsystem1 ==
  Frequency(kHz) : Inport
  Duty(%) : Inport  Port=2
  Constant1 : Constant  Value=90E6
  Divide : Product  Inputs=*/  RndMeth=Zero  SaturateOnIntegerOverflow=on
  Gain : Gain  Gain=1000
  Gain1 : Gain  Gain=1/100
  Gain2 : Gain  Gain=0.5
  Product : Product
  Product1 : Product
  Up-Down Counter : Constant  Value=2
  Out1 : Outport
  Out2 : Outport  Port=2
  Out3 : Outport  Port=3
  wires:
  Gain2/1 -> Out3/1
  Gain1/1 -> Product1/2
  Product1/1 -> Gain2/1, Out2/1
  Duty(%)/1 -> Gain1/1
  Divide/1 -> Out1/1, Product1/1
  Constant1/1 -> Divide/1
  Frequency(kHz)/1 -> Gain/1
  Product/1 -> Divide/2
  Gain/1 -> Product/1
  Up-Down Counter/1 -> Product/2

== stateflow chart C28069_LLC_ePWM_V8_230307_PhaeShiftWorking/GetADC, FaultProtection, SoftStart  @5KHz/UpdatePWM1/SoftStart/If Action Subsystem/ReservseSoftStart1/Chart1 ==
  note: Under 5KHz, 1 = 0.0002s/cycle
      | 1000 = 0.2s per increment/decrement
  note: [Frequency_Adjusted == Resonant_Frequency]
      | will go here
  note: To initialise the frequency
  note: For increment of 110 (+-5% each DC)
      | Duty_Adjusted @ 660 = 15% Duty
      | '' @ 770 = 10% Duty
      | - - - - - - - - - - - - - - - -
      | 715 + 55 = 15% DutyCycle
      | 660 + 55 (+-2.5%DC) = ~18% DutyCycle = 1us (Minimum required)
  (default) -> (junction 47)
  (junction 47) -> (junction 62) [order 2]
  (junction 62) -> (junction 64) : {
      | First_Pass = 1;
      | Soft_Start = 1;
      | Local_counter = 1;
      | SoftStart_OK = 0;
      | Duty_Adjusted = 100;
      | }
  (junction 47) -> (junction 48) [order 1] : [PFC_OK]
  (junction 48) -> (junction 49) [order 1] : [First_Pass]
  (junction 48) -> (junction 56) [order 2] : [Soft_Start]
  (junction 56) -> (junction 58) [order 1] : [Local_counter > 600]
      | {
      | Local_counter = 0;
      | }
  (junction 58) -> (junction 74) [order 2]
  (junction 74) -> (junction 81) [order 1] : [abs(Frequency_Adjusted - Resonant_Frequency)<1]
  (junction 48) -> (junction 105) [order 4]
  (junction 49) -> (junction 60) : {
      | Frequency_Adjusted = Initial_Frequency;
      | First_Pass = 0;
      | }
  (junction 48) -> (junction 102) [order 3] : [Duty_Adjusted <= 550]
  (junction 56) -> (junction 70) [order 2] : {
      | Local_counter = Local_counter +1;
      | }
  (junction 58) -> (junction 68) [order 1] : [Frequency_Adjusted > Resonant_Frequency]
      | {
      | Frequency_Adjusted = Frequency_Adjusted - 0.1;
      | }
  (junction 74) -> (junction 76) [order 2] : [Frequency_Adjusted < Resonant_Frequency]
      |
      | {
      | Frequency_Adjusted = Frequency_Adjusted + 0.1;
      | }
  (junction 81) -> (junction 84) : {
      | SoftStart_OK = 1;
      | Soft_Start = 0;
      | %%Frequency_Adjusted = Initial_Frequency;
      | }
  (junction 102) -> (junction 105) [order 2] : {
      | Local_counter = Local_counter +1;
      | }
  (junction 105) -> (junction 51)
  (junction 102) -> (junction 108) [order 1] : [Local_counter >600]
      | {
      | Local_counter = 0;
      | }
  (junction 108) -> (junction 51) : {
      | Duty_Adjusted = Duty_Adjusted + 55;
      | }
  (junction 64) -> (junction 60)
  (junction 60) -> (junction 51)
  (junction 51) -> (junction 70)
  (junction 70) -> (junction 68)
  (junction 68) -> (junction 76)
  (junction 84) -> (junction 76)
  data: SoftStart_OK output; Duty_Adjusted output =100; PFC_OK input; Initial_Frequency input; Resonant_Frequency input; Local_counter local =1; Frequency_Adjusted output double; First_Pass local =1; Soft_Start local =1

== stateflow chart C28069_LLC_ePWM_V8_230307_PhaeShiftWorking/GetADC, FaultProtection, SoftStart  @5KHz/UpdatePWM1/SoftStart/If Action Subsystem/SoftStart1/Chart ==
  note: Verror = Vbulk_Ref_ADC_adjusted - Vbulk_ADC;
  note: Local variables
      | VbusRefTemp
      | SoftStartCnt
  (default) -> (junction 47)
  (junction 47) -> (junction 50) [order 2]
  (junction 50) -> (junction 52) : {
      | First_Pass=1;
      | Soft_Start=1;
      | SoftStartCnt=1;
      | %Debug=1;
      | }
  (junction 47) -> (junction 5) [order 1] : [PFC_OK]
  (junction 5) -> (junction 7) [order 1] : [First_Pass]
  (junction 5) -> (junction 15) [order 2] : [Soft_Start]
  (junction 15) -> (junction 18) [order 1] : [SoftStartCnt>100]
      | %% At every 5 cycles (total 1ms),
  (junction 18) -> (junction 23) [order 2] : %{Debug=Vbulk_Ref_ADC_adjusted;}
  (junction 23) -> (junction 31) : %{Debug=6;}
  (junction 31) -> (junction 55) [commented out] : [abs(VBAT_Ref_adjusted - VBAT_Ref)<1]
  (junction 7) -> (junction 10) : {
      | VBAT_Ref_adjusted = VBAT_Value;
      | %Vbulk_Ref_ADC_adjusted = Vbulk_Ref_ADC;
      | First_Pass = 0;
      | %Debug=2;
      |
      | }
  (junction 5) -> (junction 38) [order 3] : {
      | SoftStart_OK = 1;
      | %Debug=3;
      | %Vbulk_Ref_ADC_adjusted=Vbulk_Ref_ADC;
      | }
  (junction 15) -> (junction 20) [order 2] : {
      | SoftStartCnt = SoftStartCnt + 1;
      | %Debug=4;
      | }
      | %% incerase the counter first.
  (junction 18) -> (junction 64) [order 1] : [VBAT_Ref_adjusted < VBAT_Ref]
      | {VBAT_Ref_adjusted = VBAT_Ref_adjusted + 0.1;}
      | %% Increase the reference voltage
  (junction 23) -> (junction 26) [commented out] : [VBAT_Ref_adjusted > VBAT_Ref]
      | {VBAT_Ref_adjusted = VBAT_Ref_adjusted - 0.1;
      | }
      | %% Reduce the reference voltage
  (junction 31) -> (junction 33) : {
      | Soft_Start=0;
      | SoftStartCnt=0;
      | %Debug=7;
      | VBAT_Ref_adjusted=VBAT_Ref;
      | }
      | %% End soft start
  (junction 55) -> (junction 57) [commented out] : {
      | Soft_Start=0;
      | SoftStartCnt=0;
      | VBAT_Ref_adjusted=VBAT_Ref;
      | %Debug=8;
      | }
  (junction 64) -> (junction 28) [order 2]
  (junction 64) -> (junction 28) [order 1] : [VBAT_Ref_adjusted < VBAT_Value]
      | {VBAT_Ref_adjusted = VBAT_Value ;}
      | %% Increase the reference voltage
  (junction 52) -> (junction 10)
  (junction 10) -> (junction 38)
  (junction 26) -> (junction 28)
  (junction 33) -> (junction 26)
  (junction 57) -> (junction 33) [commented out]
  (junction 20) -> (junction 38)
  (junction 28) -> (junction 20)
  data: PFC_OK input; VBAT_Value input; VbusRefTemp local =0; SoftStartCnt local =0; VBAT_Ref input double; VBAT_Ref_adjusted output double =0; Vbulk_Ref_ADC_Hard_Value local =0; First_Pass1 local; First_Pass local =1; Soft_Start local =1; SoftStart_OK output

== stateflow chart C28069_LLC_ePWM_V8_230307_PhaeShiftWorking/GetADC, FaultProtection, SoftStart  @5KHz/UpdatePWM1/SoftStart/If Action Subsystem/SoftStart1/Chart1 ==
  note: Under 5KHz, 1 = 0.0002s/cycle
      | 1000 = 0.2s per increment/decrement
  note: [Frequency_Adjusted == Resonant_Frequency]
      | will go here
  note: To initialise the frequency
  (default) -> (junction 47)
  (junction 47) -> (junction 62) [order 2]
  (junction 62) -> (junction 64) : {
      | First_Pass = 1;
      | Soft_Start = 1;
      | Local_counter = 1;
      | SoftStart_OK = 0;
      | }
  (junction 47) -> (junction 48) [order 1] : [PFC_OK]
  (junction 48) -> (junction 49) [order 1] : [First_Pass]
  (junction 48) -> (junction 56) [order 2] : [Soft_Start]
  (junction 56) -> (junction 58) [order 1] : [Local_counter > 400]
      | {
      | Local_counter = 0;
      | }
  (junction 58) -> (junction 74) [order 2]
  (junction 74) -> (junction 81) [order 1] : [[abs(Frequency_Adjusted - Resonant_Frequency)<1]]
  (junction 49) -> (junction 60) : {
      | Frequency_Adjusted = Initial_Frequency;
      | First_Pass = 0;
      | }
  (junction 48) -> (junction 51) [order 3]
  (junction 56) -> (junction 70) [order 2] : {
      | Local_counter = Local_counter +1;
      | }
  (junction 58) -> (junction 68) [order 1] : [Frequency_Adjusted > Resonant_Frequency]
      | {
      | Frequency_Adjusted = Frequency_Adjusted - 0.1;
      | }
  (junction 74) -> (junction 76) [order 2] : [Frequency_Adjusted < Resonant_Frequency]
      |
      | {
      | Frequency_Adjusted = Frequency_Adjusted + 0.1;
      | }
  (junction 81) -> (junction 84) : {
      | SoftStart_OK = 1;
      | Soft_Start = 0;
      | %Frequency_Adjusted = Initial_Frequency;
      | }
  (junction 64) -> (junction 60)
  (junction 60) -> (junction 51)
  (junction 51) -> (junction 70)
  (junction 70) -> (junction 68)
  (junction 68) -> (junction 76)
  (junction 84) -> (junction 76)
  data: SoftStart_OK output; PFC_OK input; Initial_Frequency input; Resonant_Frequency input; Local_counter local =1; Frequency_Adjusted output; First_Pass local =1; Soft_Start local =1

== stateflow chart C28069_LLC_ePWM_V8_230307_PhaeShiftWorking/GetADC, FaultProtection, SoftStart  @5KHz/SoftStart1/If Action Subsystem/ReservseSoftStart1/Chart1 ==
  note: Under 5KHz, 1 = 0.0002s/cycle
      | 1000 = 0.2s per increment/decrement
  note: [Frequency_Adjusted == Resonant_Frequency]
      | will go here
  note: To initialise the frequency
  note: For increment of 110 (+-5% each DC)
      | Duty_Adjusted @ 660 = 15% Duty
      | '' @ 770 = 10% Duty
      | - - - - - - - - - - - - - - - -
      | 715 + 55 = 15% DutyCycle
      | 660 + 55 (+-2.5%DC) = ~18% DutyCycle = 1us (Minimum required)
  (default) -> (junction 47)
  (junction 47) -> (junction 62) [order 2]
  (junction 62) -> (junction 64) : {
      | First_Pass = 1;
      | Soft_Start = 1;
      | Local_counter = 1;
      | SoftStart_OK = 0;
      | Duty_Adjusted = 100;
      | }
  (junction 47) -> (junction 48) [order 1] : [PFC_OK]
  (junction 48) -> (junction 49) [order 1] : [First_Pass]
  (junction 48) -> (junction 56) [order 2] : [Soft_Start]
  (junction 56) -> (junction 58) [order 1] : [Local_counter > 600]
      | {
      | Local_counter = 0;
      | }
  (junction 58) -> (junction 74) [order 2]
  (junction 74) -> (junction 81) [order 1] : [abs(Frequency_Adjusted - Resonant_Frequency)<1]
  (junction 48) -> (junction 105) [order 4]
  (junction 49) -> (junction 60) : {
      | Frequency_Adjusted = Initial_Frequency;
      | First_Pass = 0;
      | }
  (junction 48) -> (junction 102) [order 3] : [Duty_Adjusted <= 550]
  (junction 56) -> (junction 70) [order 2] : {
      | Local_counter = Local_counter +1;
      | }
  (junction 58) -> (junction 68) [order 1] : [Frequency_Adjusted > Resonant_Frequency]
      | {
      | Frequency_Adjusted = Frequency_Adjusted - 0.1;
      | }
  (junction 74) -> (junction 76) [order 2] : [Frequency_Adjusted < Resonant_Frequency]
      |
      | {
      | Frequency_Adjusted = Frequency_Adjusted + 0.1;
      | }
  (junction 81) -> (junction 84) : {
      | SoftStart_OK = 1;
      | Soft_Start = 0;
      | %%Frequency_Adjusted = Initial_Frequency;
      | }
  (junction 102) -> (junction 105) [order 2] : {
      | Local_counter = Local_counter +1;
      | }
  (junction 105) -> (junction 51)
  (junction 102) -> (junction 108) [order 1] : [Local_counter >600]
      | {
      | Local_counter = 0;
      | }
  (junction 108) -> (junction 51) : {
      | Duty_Adjusted = Duty_Adjusted + 55;
      | }
  (junction 64) -> (junction 60)
  (junction 60) -> (junction 51)
  (junction 51) -> (junction 70)
  (junction 70) -> (junction 68)
  (junction 68) -> (junction 76)
  (junction 84) -> (junction 76)
  data: SoftStart_OK output; Duty_Adjusted output =100; PFC_OK input; Initial_Frequency input; Resonant_Frequency input; Local_counter local =1; Frequency_Adjusted output double; First_Pass local =1; Soft_Start local =1

== stateflow chart C28069_LLC_ePWM_V8_230307_PhaeShiftWorking/GetADC, FaultProtection, SoftStart  @5KHz/SoftStart1/If Action Subsystem/SoftStart1/Chart ==
  note: Verror = Vbulk_Ref_ADC_adjusted - Vbulk_ADC;
  note: Local variables
      | VbusRefTemp
      | SoftStartCnt
  (default) -> (junction 47)
  (junction 47) -> (junction 50) [order 2]
  (junction 50) -> (junction 52) : {
      | First_Pass=1;
      | Soft_Start=1;
      | SoftStartCnt=1;
      | %Debug=1;
      | }
  (junction 47) -> (junction 5) [order 1] : [PFC_OK]
  (junction 5) -> (junction 7) [order 1] : [First_Pass]
  (junction 5) -> (junction 15) [order 2] : [Soft_Start]
  (junction 15) -> (junction 18) [order 1] : [SoftStartCnt>100]
      | %% At every 5 cycles (total 1ms),
  (junction 18) -> (junction 23) [order 2] : %{Debug=Vbulk_Ref_ADC_adjusted;}
  (junction 23) -> (junction 31) : %{Debug=6;}
  (junction 31) -> (junction 55) [commented out] : [abs(VBAT_Ref_adjusted - VBAT_Ref)<1]
  (junction 7) -> (junction 10) : {
      | VBAT_Ref_adjusted = VBAT_Value;
      | %Vbulk_Ref_ADC_adjusted = Vbulk_Ref_ADC;
      | First_Pass = 0;
      | %Debug=2;
      |
      | }
  (junction 5) -> (junction 38) [order 3] : {
      | SoftStart_OK = 1;
      | %Debug=3;
      | %Vbulk_Ref_ADC_adjusted=Vbulk_Ref_ADC;
      | }
  (junction 15) -> (junction 20) [order 2] : {
      | SoftStartCnt = SoftStartCnt + 1;
      | %Debug=4;
      | }
      | %% incerase the counter first.
  (junction 18) -> (junction 64) [order 1] : [VBAT_Ref_adjusted < VBAT_Ref]
      | {VBAT_Ref_adjusted = VBAT_Ref_adjusted + 0.1;}
      | %% Increase the reference voltage
  (junction 23) -> (junction 26) [commented out] : [VBAT_Ref_adjusted > VBAT_Ref]
      | {VBAT_Ref_adjusted = VBAT_Ref_adjusted - 0.1;
      | }
      | %% Reduce the reference voltage
  (junction 31) -> (junction 33) : {
      | Soft_Start=0;
      | SoftStartCnt=0;
      | %Debug=7;
      | VBAT_Ref_adjusted=VBAT_Ref;
      | }
      | %% End soft start
  (junction 55) -> (junction 57) [commented out] : {
      | Soft_Start=0;
      | SoftStartCnt=0;
      | VBAT_Ref_adjusted=VBAT_Ref;
      | %Debug=8;
      | }
  (junction 64) -> (junction 28) [order 2]
  (junction 64) -> (junction 28) [order 1] : [VBAT_Ref_adjusted < VBAT_Value]
      | {VBAT_Ref_adjusted = VBAT_Value ;}
      | %% Increase the reference voltage
  (junction 52) -> (junction 10)
  (junction 10) -> (junction 38)
  (junction 26) -> (junction 28)
  (junction 33) -> (junction 26)
  (junction 57) -> (junction 33) [commented out]
  (junction 20) -> (junction 38)
  (junction 28) -> (junction 20)
  data: PFC_OK input; VBAT_Value input; VbusRefTemp local =0; SoftStartCnt local =0; VBAT_Ref input double; VBAT_Ref_adjusted output double =0; Vbulk_Ref_ADC_Hard_Value local =0; First_Pass1 local; First_Pass local =1; Soft_Start local =1; SoftStart_OK output

== stateflow chart C28069_LLC_ePWM_V8_230307_PhaeShiftWorking/GetADC, FaultProtection, SoftStart  @5KHz/SoftStart1/If Action Subsystem/SoftStart1/Chart1 ==
  note: Under 5KHz, 1 = 0.0002s/cycle
      | 1000 = 0.2s per increment/decrement
  note: [Frequency_Adjusted == Resonant_Frequency]
      | will go here
  note: To initialise the frequency
  (default) -> (junction 47)
  (junction 47) -> (junction 62) [order 2]
  (junction 62) -> (junction 64) : {
      | First_Pass = 1;
      | Soft_Start = 1;
      | Local_counter = 1;
      | SoftStart_OK = 0;
      | }
  (junction 47) -> (junction 48) [order 1] : [PFC_OK]
  (junction 48) -> (junction 49) [order 1] : [First_Pass]
  (junction 48) -> (junction 56) [order 2] : [Soft_Start]
  (junction 56) -> (junction 58) [order 1] : [Local_counter > 400]
      | {
      | Local_counter = 0;
      | }
  (junction 58) -> (junction 74) [order 2]
  (junction 74) -> (junction 81) [order 1] : [[abs(Frequency_Adjusted - Resonant_Frequency)<1]]
  (junction 49) -> (junction 60) : {
      | Frequency_Adjusted = Initial_Frequency;
      | First_Pass = 0;
      | }
  (junction 48) -> (junction 51) [order 3]
  (junction 56) -> (junction 70) [order 2] : {
      | Local_counter = Local_counter +1;
      | }
  (junction 58) -> (junction 68) [order 1] : [Frequency_Adjusted > Resonant_Frequency]
      | {
      | Frequency_Adjusted = Frequency_Adjusted - 0.1;
      | }
  (junction 74) -> (junction 76) [order 2] : [Frequency_Adjusted < Resonant_Frequency]
      |
      | {
      | Frequency_Adjusted = Frequency_Adjusted + 0.1;
      | }
  (junction 81) -> (junction 84) : {
      | SoftStart_OK = 1;
      | Soft_Start = 0;
      | %Frequency_Adjusted = Initial_Frequency;
      | }
  (junction 64) -> (junction 60)
  (junction 60) -> (junction 51)
  (junction 51) -> (junction 70)
  (junction 70) -> (junction 68)
  (junction 68) -> (junction 76)
  (junction 84) -> (junction 76)
  data: SoftStart_OK output; PFC_OK input; Initial_Frequency input; Resonant_Frequency input; Local_counter local =1; Frequency_Adjusted output; First_Pass local =1; Soft_Start local =1

== stateflow chart C28069_LLC_ePWM_V8_230307_PhaeShiftWorking/GetADC, FaultProtection, SoftStart  @5KHz/SoftStart1/ReservseSoftStart/Chart1 ==
  note: Under 5KHz, 1 = 0.0002s/cycle
      | 1000 = 0.2s per increment/decrement
  note: [Frequency_Adjusted == Resonant_Frequency]
      | will go here
  note: To initialise the frequency
  note: For increment of 110 (+-5% each DC)
      | Duty_Adjusted @ 660 = 15% Duty
      | '' @ 770 = 10% Duty
      | - - - - - - - - - - - - - - - -
      | 715 + 55 = 15% DutyCycle
      | 660 + 55 (+-2.5%DC) = ~18% DutyCycle = 1us (Minimum required)
  (default) -> (junction 47)
  (junction 47) -> (junction 62) [order 2]
  (junction 62) -> (junction 64) : {
      | First_Pass = 1;
      | Soft_Start = 1;
      | Local_counter = 1;
      | SoftStart_OK = 0;
      | Duty_Adjusted = 100;
      | }
  (junction 47) -> (junction 48) [order 1] : [PFC_OK]
  (junction 48) -> (junction 49) [order 1] : [First_Pass]
  (junction 48) -> (junction 56) [order 2] : [Soft_Start]
  (junction 56) -> (junction 58) [order 1] : [Local_counter > 600]
      | {
      | Local_counter = 0;
      | }
  (junction 58) -> (junction 74) [order 2]
  (junction 74) -> (junction 81) [order 1] : [abs(Frequency_Adjusted - Resonant_Frequency)<1]
  (junction 48) -> (junction 105) [order 4]
  (junction 49) -> (junction 60) : {
      | Frequency_Adjusted = Initial_Frequency;
      | First_Pass = 0;
      | }
  (junction 48) -> (junction 102) [order 3] : [Duty_Adjusted <= 550]
  (junction 56) -> (junction 70) [order 2] : {
      | Local_counter = Local_counter +1;
      | }
  (junction 58) -> (junction 68) [order 1] : [Frequency_Adjusted > Resonant_Frequency]
      | {
      | Frequency_Adjusted = Frequency_Adjusted - 0.1;
      | }
  (junction 74) -> (junction 76) [order 2] : [Frequency_Adjusted < Resonant_Frequency]
      |
      | {
      | Frequency_Adjusted = Frequency_Adjusted + 0.1;
      | }
  (junction 81) -> (junction 84) : {
      | SoftStart_OK = 1;
      | Soft_Start = 0;
      | %%Frequency_Adjusted = Initial_Frequency;
      | }
  (junction 102) -> (junction 105) [order 2] : {
      | Local_counter = Local_counter +1;
      | }
  (junction 105) -> (junction 51)
  (junction 102) -> (junction 108) [order 1] : [Local_counter >600]
      | {
      | Local_counter = 0;
      | }
  (junction 108) -> (junction 51) : {
      | Duty_Adjusted = Duty_Adjusted + 55;
      | }
  (junction 64) -> (junction 60)
  (junction 60) -> (junction 51)
  (junction 51) -> (junction 70)
  (junction 70) -> (junction 68)
  (junction 68) -> (junction 76)
  (junction 84) -> (junction 76)
  data: SoftStart_OK output; Duty_Adjusted output =100; PFC_OK input; Initial_Frequency input; Resonant_Frequency input; Local_counter local =1; Frequency_Adjusted output double; First_Pass local =1; Soft_Start local =1

== stateflow chart C28069_LLC_ePWM_V8_230307_PhaeShiftWorking/GetADC, FaultProtection, SoftStart  @5KHz/SoftStart1/SoftStart/Chart ==
  note: Verror = Vbulk_Ref_ADC_adjusted - Vbulk_ADC;
  note: Local variables
      | VbusRefTemp
      | SoftStartCnt
  (default) -> (junction 47)
  (junction 47) -> (junction 50) [order 2]
  (junction 50) -> (junction 52) : {
      | First_Pass=1;
      | Soft_Start=1;
      | SoftStartCnt=1;
      | %Debug=1;
      | }
  (junction 47) -> (junction 5) [order 1] : [PFC_OK]
  (junction 5) -> (junction 7) [order 1] : [First_Pass]
  (junction 5) -> (junction 15) [order 2] : [Soft_Start]
  (junction 15) -> (junction 18) [order 1] : [SoftStartCnt>100]
      | %% At every 5 cycles (total 1ms),
  (junction 18) -> (junction 23) [order 2] : %{Debug=Vbulk_Ref_ADC_adjusted;}
  (junction 23) -> (junction 31) [order 2] : %{Debug=6;}
  (junction 31) -> (junction 55) [order 1] : [abs(VBAT_Ref_adjusted - VBAT_Ref)<1]
  (junction 7) -> (junction 10) : {
      | VBAT_Ref_adjusted = VBAT_Value;
      | %Vbulk_Ref_ADC_adjusted = Vbulk_Ref_ADC;
      | First_Pass = 0;
      | %Debug=2;
      |
      | }
  (junction 5) -> (junction 38) [order 3] : {
      | %Debug=3;
      | %Vbulk_Ref_ADC_adjusted=Vbulk_Ref_ADC;
      | }
  (junction 15) -> (junction 20) [order 2] : {
      | SoftStartCnt = SoftStartCnt + 1;
      | %Debug=4;
      | }
      | %% incerase the counter first.
  (junction 18) -> (junction 64) [order 1] : [VBAT_Ref_adjusted < VBAT_Ref]
      | {VBAT_Ref_adjusted = VBAT_Ref_adjusted + 0.1;}
      | %% Increase the reference voltage
  (junction 23) -> (junction 26) [order 1] : [VBAT_Ref_adjusted > VBAT_Ref]
      | {VBAT_Ref_adjusted = VBAT_Ref_adjusted - 0.1;
      | }
      | %% Reduce the reference voltage
  (junction 31) -> (junction 33) [order 2] : {
      | Soft_Start=0;
      | SoftStartCnt=0;
      | %Debug=7;
      | }
      | %% End soft start
  (junction 55) -> (junction 57) : {
      | Soft_Start=0;
      | SoftStartCnt=0;
      | VBAT_Ref_adjusted=VBAT_Ref;
      | %Debug=8;
      | }
  (junction 64) -> (junction 28) [order 2]
  (junction 64) -> (junction 28) [order 1] : [VBAT_Ref_adjusted < VBAT_Value]
      | {VBAT_Ref_adjusted = VBAT_Value ;}
      | %% Increase the reference voltage
  (junction 52) -> (junction 10)
  (junction 10) -> (junction 38)
  (junction 26) -> (junction 28)
  (junction 33) -> (junction 26)
  (junction 57) -> (junction 33)
  (junction 20) -> (junction 38)
  (junction 28) -> (junction 20)
  data: PFC_OK input; VBAT_Value input; VbusRefTemp local =0; SoftStartCnt local =0; VBAT_Ref input double; VBAT_Ref_adjusted output double =0; Vbulk_Ref_ADC_Hard_Value local =0; First_Pass1 local; First_Pass local =1; Soft_Start local =1

== stateflow chart C28069_LLC_ePWM_V8_230307_PhaeShiftWorking/GetADC, FaultProtection, SoftStart  @5KHz/SoftStart1/SoftStart/Chart1 ==
  note: Under 5KHz, 1 = 0.0002s/cycle
      | 1000 = 0.2s per increment/decrement
  note: [Frequency_Adjusted == Resonant_Frequency]
      | will go here
  note: To initialise the frequency
  (default) -> (junction 47)
  (junction 47) -> (junction 62) [order 2]
  (junction 62) -> (junction 64) : {
      | First_Pass = 1;
      | Soft_Start = 1;
      | Local_counter = 1;
      | SoftStart_OK = 0;
      | }
  (junction 47) -> (junction 48) [order 1] : [PFC_OK]
  (junction 48) -> (junction 49) [order 1] : [First_Pass]
  (junction 48) -> (junction 56) [order 2] : [Soft_Start]
  (junction 56) -> (junction 58) [order 1] : [Local_counter > 400]
      | {
      | Local_counter = 0;
      | }
  (junction 58) -> (junction 74) [order 2]
  (junction 74) -> (junction 81) [order 1] : [[abs(Frequency_Adjusted - Resonant_Frequency)<1]]
  (junction 49) -> (junction 60) : {
      | Frequency_Adjusted = Initial_Frequency;
      | First_Pass = 0;
      | }
  (junction 48) -> (junction 51) [order 3]
  (junction 56) -> (junction 70) [order 2] : {
      | Local_counter = Local_counter +1;
      | }
  (junction 58) -> (junction 68) [order 1] : [Frequency_Adjusted > Resonant_Frequency]
      | {
      | Frequency_Adjusted = Frequency_Adjusted - 0.1;
      | }
  (junction 74) -> (junction 76) [order 2] : [Frequency_Adjusted < Resonant_Frequency]
      |
      | {
      | Frequency_Adjusted = Frequency_Adjusted + 0.1;
      | }
  (junction 81) -> (junction 84) : {
      | SoftStart_OK = 1;
      | Soft_Start = 0;
      | %Frequency_Adjusted = Initial_Frequency;
      | }
  (junction 64) -> (junction 60)
  (junction 60) -> (junction 51)
  (junction 51) -> (junction 70)
  (junction 70) -> (junction 68)
  (junction 68) -> (junction 76)
  (junction 84) -> (junction 76)
  data: SoftStart_OK output; PFC_OK input; Initial_Frequency input; Resonant_Frequency input; Local_counter local =1; Frequency_Adjusted output; First_Pass local =1; Soft_Start local =1
